simulink library "PV_Generator"  (Simulink 8.2)
settings: Solver=ode45  StartTime=0.0  StopTime=10.0  RelTol=1e-3
libraries: carnot x2
settings Model: Creator=lena.frank  LastModifiedBy=drhf

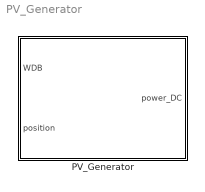
== system PV_Generator ==
  PV_Generator : Subsystem  mask(PV_Module_simple){Wp=1000, delta_Wp_K=0.0047, fgen=0.91 % 0.06 power missmatch, 0.01 diodes, 0.02 data sheet tolerance}
      mask prompts: Wp "Peak power of the generator [W]"; delta_Wp_K "Temperature coefficient Pmax 1/K"; fgen "efficiency generator field (lossses in diodes, power missmatch, dirt)"
      mask help:
      | This block simultes a pv panel and calculates the output of the module in Ws based on the parameters
      | - Wp of one panel at STC [W]
      | - temperature coefficient of Pmax [1/K]
      | - number of panels [1]
      |
      | Input
      | - weather inclined
      |
      | Output
      | - DC power of the PV generator
      mask Help: web(fullfile(path_carnot('help'),'PV_Generator.html'),'-helpbrowser')
      mask Display: plot(0,0,100,100,[10,40,90,60,10],[10,90,90,10,10],[37,53,60,43,37],[70,70,86,86,70],[60,75,82,67,60],[70,71,86,86,70],[35,30,43,51,35],[65,50,49,65,65],[51,67,73,58,51],[50,50,66,66,50],[28,20,36,43,28],[41,23,23,41,41],[49,44,58,65,49],[41,23,22,41,41])

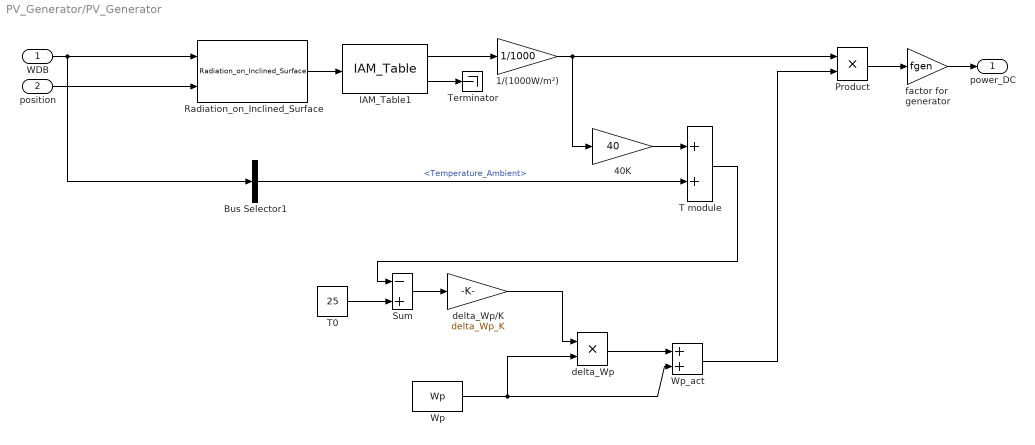
== system PV_Generator/PV_Generator ==
  WDB : Inport
  position : Inport  Port=2
  1/(1000W/m²) : Gain  Gain=1/1000
  40K : Gain  Gain=40
  Bus Selector1 : BusSelector  OutputSignals=Temperature_Ambient
  IAM_Table1 : carnot/Source/Solar_Thermal/IncidenceAngleModifier/IAM_Table  angle=[0:5:90]  Kb="[1.0000    1.0000    0.9999    0.9996    0.9991    0.9982    0.9965  0.9935    0.9886    0.9807    0.9678    0.9473    0.9148    0.8638   0.7846    0.6644    0.4907    0.2599    0.0000]"  Kd=0.915  fta=1
  Product : Product  RndMeth=Zero
  Radiation_on_Inclined_Surface : carnot/Weather/Radiation_on_Inclined_Surface  sky=Perez 1990  reflect=0.2
  Sum : Sum  Inputs=-+
  T module : Sum  Inputs=2
  T0 : Constant  Value=25
  Terminator : Terminator
  Wp : Constant  Value=Wp
  Wp_act : Sum
  delta_Wp : Product  RndMeth=Zero
  delta_Wp/K : Gain  Gain=delta_Wp_K
  factor for  generator : Gain  Gain=fgen
  power_DC : Outport
  wires:
  delta_Wp/1 -> Wp_act/1
  Wp/1 -> Wp_act/2, delta_Wp/2
  Bus Selector1/1 -> T module/2  "<Temperature_Ambient>"
  40K/1 -> T module/1
  Sum/1 -> delta_Wp/K/1
  T0/1 -> Sum/2
  IAM_Table1/1 -> 1/(1000W/m²)/1
  T module/1 -> Sum/1
  Wp_act/1 -> Product/2
  1/(1000W/m²)/1 -> 40K/1, Product/1
  Product/1 -> factor for  generator/1
  delta_Wp/K/1 -> delta_Wp/1
  factor for  generator/1 -> power_DC/1
  WDB/1 -> Bus Selector1/1, Radiation_on_Inclined_Surface/1
  Radiation_on_Inclined_Surface/1 -> IAM_Table1/1
  position/1 -> Radiation_on_Inclined_Surface/2
  IAM_Table1/2 -> Terminator/1
